simulink model "sra3"  (R2016a)
settings: Solver=ode45  StartTime=0.0  StopTime=30  RelTol=1e-5
values from neighbouring files (symbols this model uses):
  R_cu = conv([1 b], [1 -1])    [program3.m]
  R_fara = conv([1 -1], [1 X(4)])    [program3.m]
  S_cu = [(p1-a1+1)/K (p0-a0+a1)/K a0/K]    [program3.m]
  S_fara = X(1:3)'    [program3.m]
  T_cu = conv([1 0], [(1+p1+p0) 0])/K    [program3.m]
  T_fara = conv([1 0 0], (1+p1+p0)/K/(1+b))    [program3.m]
  Te = 0.01    [program3.m]
libraries: simulink x2
settings Model: Creator=andrei  LastModifiedBy=andrei

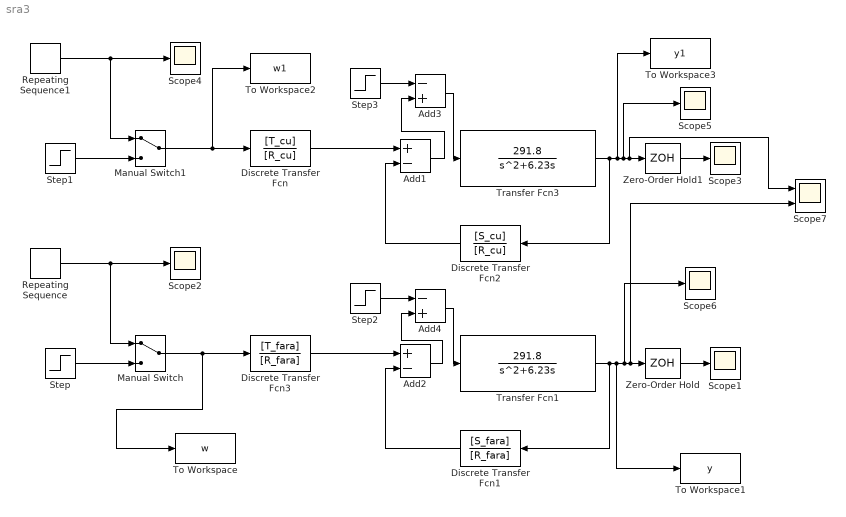
== system sra3 ==
  Add1 : Sum  Inputs=+-
  Add2 : Sum  Inputs=+-
  Add3 : Sum  Inputs=-+
  Add4 : Sum  Inputs=-+
  Discrete Transfer Fcn : DiscreteTransferFcn  Numerator=[T_cu]  Denominator=[R_cu]  SampleTime=Te
  Discrete Transfer Fcn1 : DiscreteTransferFcn  Numerator=[S_fara]  Denominator=[R_fara]  SampleTime=Te
  Discrete Transfer Fcn2 : DiscreteTransferFcn  Numerator=[S_cu]  Denominator=[R_cu]  SampleTime=Te
  Discrete Transfer Fcn3 : DiscreteTransferFcn  Numerator=[T_fara]  Denominator=[R_fara]  SampleTime=Te
  Manual Switch : ManualSwitch
  Manual Switch1 : ManualSwitch
  Repeating Sequence : simulink/Sources/Repeating Sequence  rep_seq_t=[0.0001 5 5.0001 10 10.0001]  rep_seq_y=[0.0001 0.0000 5 5 5]
  Repeating Sequence1 : simulink/Sources/Repeating Sequence  rep_seq_t=[0.0001 5 5.0001 10 10.0001]  rep_seq_y=[0.0001 0.0000 5 5 5]
  Scope{1..6} (6 alike) : Scope
  Scope7 : Scope  NumInputPorts=2
  Step : Step  Time=0  SampleTime=0
  Step1 : Step  Time=0  SampleTime=0
  Step2 : Step  Time=7.5  After=0.01  SampleTime=0
  Step3 : Step  Time=7.5  After=0.01  SampleTime=0
  To Workspace : ToWorkspace  VariableName=w  SaveFormat=Timeseries  SampleTime=-1
  To Workspace1 : ToWorkspace  VariableName=y  SaveFormat=Timeseries  SampleTime=-1
  To Workspace2 : ToWorkspace  VariableName=w1  SaveFormat=Timeseries  SampleTime=-1
  To Workspace3 : ToWorkspace  VariableName=y1  SaveFormat=Timeseries  SampleTime=-1
  Transfer Fcn1 : TransferFcn  Numerator=[291.8]  Denominator=[1 6.23 0]
  Transfer Fcn3 : TransferFcn  Numerator=[291.8]  Denominator=[1 6.23 0]
  Zero-Order Hold : ZeroOrderHold  SampleTime=Te
  Zero-Order Hold1 : ZeroOrderHold  SampleTime=Te
  wires:
  Repeating Sequence/1 -> Manual Switch/1, Scope2/1
  Step/1 -> Manual Switch/2
  Discrete Transfer Fcn3/1 -> Add2/1
  Discrete Transfer Fcn1/1 -> Add2/2
  Transfer Fcn1/1 -> To Workspace1/1, Scope6/1, Scope7/2, Zero-Order Hold/1, Discrete Transfer Fcn1/1
  Zero-Order Hold/1 -> Scope1/1
  Repeating Sequence1/1 -> Manual Switch1/1, Scope4/1
  Step1/1 -> Manual Switch1/2
  Manual Switch1/1 -> To Workspace2/1, Discrete Transfer Fcn/1
  Discrete Transfer Fcn/1 -> Add1/1
  Discrete Transfer Fcn2/1 -> Add1/2
  Transfer Fcn3/1 -> To Workspace3/1, Scope5/1, Scope7/1, Zero-Order Hold1/1, Discrete Transfer Fcn2/1
  Zero-Order Hold1/1 -> Scope3/1
  Manual Switch/1 -> To Workspace/1, Discrete Transfer Fcn3/1
  Step3/1 -> Add3/1
  Add1/1 -> Add3/2
  Add3/1 -> Transfer Fcn3/1
  Step2/1 -> Add4/1
  Add2/1 -> Add4/2
  Add4/1 -> Transfer Fcn1/1
